simulink model "dcdc_joint"  (R2020b)
settings: Solver=VariableStepAuto  StartTime=0.0  StopTime=0.4  FixedStep=t_step  MaxStep=1e-6  RelTol=1e-3
undefined symbols (not defined in the file): Cb, Ion, Lb, Lithium, t_step
libraries: powerlib x19, powerlib_meascontrol x5, electricdrivelib x1
settings Model: Creator=Chuanyue Li  LastModifiedBy=c2107789
settings SolverCC: ZeroCrossAlgorithm=Adaptive
settings DataIOCC: ReturnWorkspaceOutputs=off
settings DebuggingCC: IgnoredZcDiagnostic=none  ArithmeticOperatorsInVariantConditions=warning
settings SFSimCC: SimUseLocalCustomCode=off  CustomCodeUndefinedFunction=UseInterfaceOnly
settings RTWCC: RTWUseLocalCustomCode=off

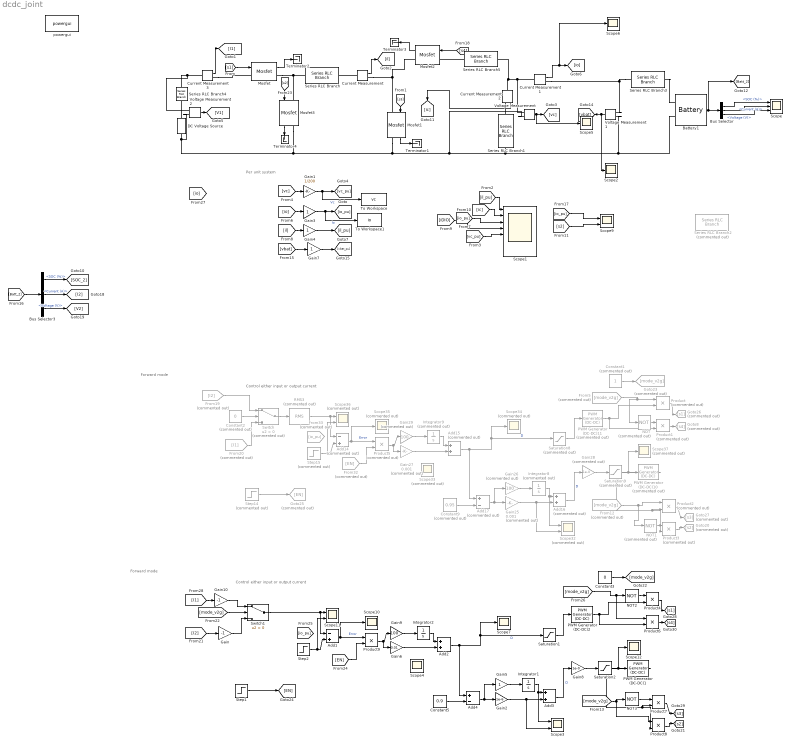
== system dcdc_joint ==
  note: Control either input or output current
  note: Per unit system
  note: Forward mode
  note: Control either input or output current
  note: Forward mode
  Add1 : Sum  Inputs=-+
  Add14 : Sum  Commented=on  Inputs=-+
  Add15 : Sum  Commented=on
  Add16 : Sum  Commented=on
  Add17 : Sum  Commented=on  Inputs=+-
  Add2 : Sum
  Add3 : Sum
  Add4 : Sum  Inputs=+-
  Battery1 : electricdrivelib/Extra Sources/Battery  BatType=Lithium-Ion  ShowTempParam=off  ThermalPreset=no  ShowAgeParam=off  NomV=380  NomQ=500  SOC=69.98  Batt_Tr=1  PresetModel=on  MaxQ=500  MinV=285  FullV=442.3151  Dis_rate=217.3913  R=0.0076  Normal_OP=452.1739  expZone="[410.5466      24.56522]"  current=[6.5 13 32.5]  Units=Time  Tci=20  NomT=20  T2=-30  MaxQ2=4.8  FullV2=7.1  Normal_OP2=5.655  expZone2="[6.58           1]"  Rca=0.6  ti=2000  Dp=0  Neq0=0  Tsim=1e6  Ta1=25  Qeol=5.4*0.9  Reol=0.013333*1.2  Char_age=[2.3478, 3]  Dis_age=[2.3478, 10]  N1=1500  N2=10500  N3=1000  N4=1400  Ta2=45  N5=950
  Bus Selector : BusSelector  OutputSignals=SOC (%),Current (A),Voltage (V)
  Bus Selector3 : BusSelector  OutputSignals=SOC (%),Current (A),Voltage (V)
  Constant1 : Constant  Commented=on
  Constant2 : Constant  Commented=on  Value=0
  Constant3 : Constant  Value=0
  Constant5 : Constant  Value=0.9
  Constant9 : Constant  Commented=on  Value=0.95
  Current Measurement{,1..3} (4 alike) : powerlib/Measurements/Current Measurement  PhasorSimulation=off  OutputType=Complex  PSBequivalent=0
  DC Voltage Source : powerlib/Electrical Sources/DC Voltage Source  Amplitude=415  Measurements=None
  From12 : From  Commented=on  GotoTag=mode_v2g
  From19 : From  Commented=on  GotoTag=I2
  From20 : From  Commented=on  GotoTag=I1
  From32 : From  Commented=on  GotoTag=EN
  From33 : From  Commented=on  GotoTag=io_pu
  From5 : From  Commented=on  GotoTag=mode_v2g
  Gain : Gain  Gain=-1
  Gain1 : Gain  Gain=1/200
  Gain10 : Gain  Gain=-1
  Gain2 : Gain  Gain=1e-6
  Gain25 : Gain  Commented=on  Gain=0.001
  Gain26 : Gain  Commented=on  Gain=100
  Gain27 : Gain  Commented=on  Gain=0.001
  Gain28 : Gain  Commented=on  Gain=1e-0
  Gain29 : Gain  Commented=on  Gain=100
  Gain{3..5,7} (4 alike) : Gain
  Gain6 : Gain  Gain=0.01
  Gain8 : Gain  Gain=1e-0
  Gain9 : Gain  Gain=100
  Goto20 : Goto  Commented=on  GotoTag=s2
  Goto23 : Goto  Commented=on  GotoTag=mode_v2g
  Goto25 : Goto  Commented=on  GotoTag=EN
  Goto26 : Goto  Commented=on  GotoTag=s1
  Goto27 : Goto  Commented=on  GotoTag=s3
  Goto8 : Goto  Commented=on  GotoTag=s4
  Integrator1 : Integrator  LimitOutput=on  UpperSaturationLimit=1  LowerSaturationLimit=0
  Integrator2 : Integrator  LimitOutput=on  UpperSaturationLimit=2  LowerSaturationLimit=0
  Integrator8 : Integrator  Commented=on  LimitOutput=on  UpperSaturationLimit=1  LowerSaturationLimit=0
  Integrator9 : Integrator  Commented=on  LimitOutput=on  UpperSaturationLimit=2  LowerSaturationLimit=0
  Mosfet : powerlib/Power Electronics/Mosfet  Ron=0.1  Lon=0  Rd=0.01  Vfd=0  IC=0  Rs=1e5  Cs=inf  Measurements=on
  Mosfet1 : powerlib/Power Electronics/Mosfet  Ron=0.01  Lon=0  Rd=0.01  Vfd=0  IC=0  Rs=1e5  Cs=inf  Measurements=on
  Mosfet2 : powerlib/Power Electronics/Mosfet  Ron=0.1  Lon=0  Rd=0.01  Vfd=0  IC=0  Rs=1e5  Cs=inf  Measurements=on
  Mosfet3 : powerlib/Power Electronics/Mosfet  Ron=0.1  Lon=0  Rd=0.01  Vfd=0  IC=0  Rs=1e5  Cs=inf  Measurements=on
  NOT : Logic  Commented=on  Operator=NOT  IconShape=distinctive  AllPortsSameDT=off  OutDataTypeStr=boolean
  NOT1 : Logic  Commented=on  Operator=NOT  IconShape=distinctive  AllPortsSameDT=off  OutDataTypeStr=boolean
  NOT2 : Logic  Operator=NOT  IconShape=distinctive  AllPortsSameDT=off  OutDataTypeStr=boolean
  NOT3 : Logic  Operator=NOT  IconShape=distinctive  AllPortsSameDT=off  OutDataTypeStr=boolean
  PWM Generator (DC-DC)1 : powerlib_meascontrol/Pulse & Signal Generators/PWM Generator (DC-DC)  Fsw=s_fre  Ts=0
  PWM Generator (DC-DC)10 : powerlib_meascontrol/Pulse & Signal Generators/PWM Generator (DC-DC)  Commented=on  Fsw=s_fre  Ts=0
  PWM Generator (DC-DC)11 : powerlib_meascontrol/Pulse & Signal Generators/PWM Generator (DC-DC)  Commented=on  Fsw=s_fre  Ts=0
  PWM Generator (DC-DC)2 : powerlib_meascontrol/Pulse & Signal Generators/PWM Generator (DC-DC)  Fsw=s_fre  Ts=0
  Product{,1..3,5} (5 alike) : Product  Commented=on
  Product{4,6..9} (5 alike) : Product
  RMS3 : powerlib_meascontrol/Measurements/RMS  Commented=on  TrueRMS=on  Freq=s_fre  RMSInit=0  Ts=0
  Saturation1 : Saturate  UpperLimit=1  LowerLimit=0
  Saturation2 : Saturate  UpperLimit=0.8  LowerLimit=0
  Saturation8 : Saturate  Commented=on  UpperLimit=1  LowerLimit=0
  Saturation9 : Saturate  Commented=on  UpperLimit=0.8  LowerLimit=0
  Scope : Scope  NumInputPorts=3
  Scope1 : Scope  NumInputPorts=8
  Scope{2,4..7,10,12} (7 alike) : Scope
  Scope11 : Scope  NumInputPorts=2
  Scope3 : Scope  NumInputPorts=2
  Scope32 : Scope  Commented=on  NumInputPorts=2
  Scope{33..35,37} (4 alike) : Scope  Commented=on
  Scope36 : Scope  Commented=on  NumInputPorts=2
  Scope9 : Scope  NumInputPorts=2
  Series RLC Branch : powerlib/Elements/Series RLC Branch  LConnTagsString=__new0  RConnTagsString=__new0  BranchType=L  Resistance=1  Inductance=Lb/100  SetiL0=off  InitialCurrent=0  Capacitance=1e-6  Setx0=off  InitialVoltage=0  Measurements=None
  Series RLC Branch1 : powerlib/Elements/Series RLC Branch  LConnTagsString=__new0  RConnTagsString=__new0  BranchType=C  Resistance=1  Inductance=1e-3  SetiL0=off  InitialCurrent=0  Capacitance=Cb  Setx0=off  InitialVoltage=0  Measurements=None
  Series RLC Branch2 : powerlib/Elements/Series RLC Branch  Commented=on  LConnTagsString=__new0  RConnTagsString=__new0  BranchType=L  Resistance=1  Inductance=Lb/100  SetiL0=off  InitialCurrent=0  Capacitance=1e-6  Setx0=off  InitialVoltage=0  Measurements=None
  Series RLC Branch3 : powerlib/Elements/Series RLC Branch  LConnTagsString=__new0  RConnTagsString=__new0  BranchType=R  Resistance=1  Inductance=Lb/100  SetiL0=off  InitialCurrent=0  Capacitance=1e-6  Setx0=off  InitialVoltage=0  Measurements=None
  Series RLC Branch4 : powerlib/Elements/Series RLC Branch  LConnTagsString=__new0  RConnTagsString=__new0  BranchType=R  Resistance=1e-3  Inductance=1e-3  SetiL0=off  InitialCurrent=0  Capacitance=Cb  Setx0=off  InitialVoltage=0  Measurements=None
  Series RLC Branch5 : powerlib/Elements/Series RLC Branch  LConnTagsString=__new0  RConnTagsString=__new0  BranchType=L  Resistance=1  Inductance=Lb/100  SetiL0=off  InitialCurrent=0  Capacitance=1e-6  Setx0=off  InitialVoltage=0  Measurements=None
  Step1 : Step  Time=0.025  SampleTime=0
  Step14 : Step  Commented=on  Time=0.025  SampleTime=0
  Step15 : Step  Commented=on  Before=10  After=11  SampleTime=0
  Step2 : Step  Before=30  After=11  SampleTime=0
  Switch : Switch  Commented=on  Criteria=u2 > Threshold
  Switch1 : Switch  Criteria=u2 > Threshold
  Terminator{1..4} (4 alike) : Terminator
  To Workspace : ToWorkspace  VariableName=vc  SaveFormat=Timeseries  SampleTime=-1
  To Workspace1 : ToWorkspace  VariableName=io  SaveFormat=Timeseries  SampleTime=-1
  Voltage Measurement : powerlib/Measurements/Voltage Measurement  PhasorSimulation=off  OutputType=Complex  PSBequivalent=0
  Voltage Measurement1 : powerlib/Measurements/Voltage Measurement  PhasorSimulation=off  OutputType=Complex  PSBequivalent=0
  Voltage Measurement2 : powerlib/Measurements/Voltage Measurement  PhasorSimulation=off  OutputType=Complex  PSBequivalent=0
  powergui : powerlib/powergui  Priority=1  SimulationMode=Continuous  SampleTime=t_step*10  frequency=60  Iterations=50  frequencyindice=0  Pbase=100e6  ErrMax=1e-4  UnitsV=kV  UnitsW=MW  buscounter=0  FunctionMessages=off  echomessages=off  EnableUseOfTLC=off  CurrentSourceSwitches=off  DisableSnubberDevices=off  DisableRonSwitches=off  DisableVfSwitches=off  DisplayEquations=off  AutomaticDiscreteSolvers=off  SolverType=Tustin/Backward Euler (TBE)  Interpol=off  ExternalGateDelay=off  methode=off  Ts=100  x0status=blocks  SPID=off  SwTol=0  HookPort=off  NonlinearTolerance=1e-4  nMaxIteration=100  ContinueOnMaxIteration=off  RestoreLinks=warning  ResistiveCurrentMeasurement=off  Frange=[0:2:500]  Ylog=off  Xlog=on  ShowGrid=off  save=off  variable=ZData  structure=0  ZoomFFT=off  StartTime=0.0  cycles=1  DisplayStyle=1  fundamental=60  FreqAxis=off  MaxFrequency=1000  frequencyindicesteady=1  RmsSteady=1  display=off
  wires:
  [s1] -> Mosfet/1
  [s3] -> Mosfet1/1
  Current Measurement/1 -> [il]
  Voltage Measurement/1 -> Scope5/1, [vc]
  [il_pu] -> Scope1/1
  [vc] -> Gain1/1
  Gain1/1 -> To Workspace/1, [vc_pu]  "Vc"
  Bus Selector/1 -> Scope/1  "<SOC (%)>"
  Bus Selector/2 -> Scope/2  "<Current (A)>"
  Bus Selector/3 -> Scope/3  "<Voltage (V)>"
  [io] -> Gain3/1
  Current Measurement1/1 -> Scope6/1, [io]
  Gain3/1 -> To Workspace1/1, [io_pu]  "Io"
  [io_pu] -> Scope1/3
  Gain4/1 -> [il_pu]
  [il] -> Gain4/1
  [iDIO] -> Scope1/4
  Current Measurement2/1 -> [ic]
  [ic] -> Scope1/2
  [vc_pu] -> Scope1/5
  Voltage Measurement1/1 -> Scope2/1, [vbat]
  [vbat] -> Gain7/1
  Gain7/1 -> [vbat_pu]
  Mosfet1/1 -> Terminator1/1
  Mosfet/1 -> Terminator2/1
  [io_pu] -> Scope9/1
  [s2] -> Scope9/2
  Mosfet2/1 -> Terminator3/1
  [s4] -> Mosfet2/1
  [s2] -> Mosfet3/1
  Mosfet3/1 -> Terminator4/1
  Add16/1 -> Gain28/1  "D"
  Gain26/1 -> Integrator8/1
  Gain25/1 -> Add16/2, Scope32/2
  Integrator8/1 -> Add16/1, Scope32/1
  Saturation8/1 -> PWM Generator (DC-DC)11/1
  Integrator9/1 -> Add15/1
  Add15/1 -> Saturation8/1, Scope34/1, Add17/1  "D"
  From32/1 -> Product5/2
  Product5/1 -> Gain29/1, Gain27/1
  Step14/1 -> Goto25/1
  Gain27/1 -> Add15/2
  Gain29/1 -> Integrator9/1
  Step15/1 -> Scope36/2, Add14/2
  Add14/1 -> Product5/1, Scope35/1  "Error"
  Saturation9/1 -> PWM Generator (DC-DC)10/1, Scope37/1
  Switch/1 -> RMS3/1
  PWM Generator (DC-DC)11/1 -> Product/2, Product1/2
  Gain28/1 -> Saturation9/1
  Constant9/1 -> Add17/2
  Add17/1 -> Gain25/1, Gain26/1
  Battery1/1 -> [Batt_2], Bus Selector/1
  [Batt_2] -> Bus Selector3/1
  Bus Selector3/3 -> [V2]  "<Voltage (V)>"
  Bus Selector3/2 -> [I2]  "<Current (A)>"
  Bus Selector3/1 -> [SOC_2]  "<SOC (%)>"
  From19/1 -> Switch/1
  From20/1 -> Switch/3
  Constant2/1 -> Switch/2
  Product/1 -> Goto26/1
  Product1/1 -> Goto8/1
  NOT/1 -> Product1/1
  NOT1/1 -> Product3/1
  Product3/1 -> Goto20/1
  From12/1 -> NOT1/1, Product2/1
  Product2/1 -> Goto27/1
  PWM Generator (DC-DC)10/1 -> Product3/2, Product2/2
  Constant1/1 -> Goto23/1
  From5/1 -> Product/1, NOT/1
  Current Measurement3/1 -> [I1]
  Voltage Measurement2/1 -> [V1]
  RMS3/1 -> Add14/1, Scope36/1
  Switch1/1 -> Scope11/1, Add1/1
  Constant3/1 -> [mode_v2g]
  PWM Generator (DC-DC)1/1 -> Product7/2, Product8/2
  Product7/1 -> [s3]
  Product8/1 -> [s2]
  [mode_v2g] -> Product8/1, NOT3/1
  [mode_v2g] -> NOT2/1, Product6/1
  Product6/1 -> [s4]
  Product4/1 -> [s1]
  [mode_v2g] -> Switch1/2
  [I2] -> Gain/1
  Add4/1 -> Gain5/1, Gain2/1
  Constant5/1 -> Add4/2
  Gain8/1 -> Saturation2/1
  PWM Generator (DC-DC)2/1 -> Product6/2, Product4/2
  Saturation2/1 -> Scope12/1, PWM Generator (DC-DC)1/1
  Add1/1 -> Scope10/1, Product9/1  "Error"
  Step2/1 -> Add1/2, Scope11/2
  Gain9/1 -> Integrator2/1
  Gain6/1 -> Add2/2
  Step1/1 -> [EN]
  Product9/1 -> Gain6/1, Gain9/1
  [EN] -> Product9/2
  Add2/1 -> Add4/1, Scope7/1, Saturation1/1  "D"
  Integrator2/1 -> Add2/1
  Saturation1/1 -> PWM Generator (DC-DC)2/1
  Integrator1/1 -> Scope3/1, Add3/1
  Gain2/1 -> Scope3/2, Add3/2
  Gain5/1 -> Integrator1/1
  Add3/1 -> Gain8/1  "D"
  NOT2/1 -> Product4/1
  NOT3/1 -> Product7/1
  Gain/1 -> Switch1/3
  Gain10/1 -> Switch1/1
  [I1] -> Gain10/1
  connections:
  Mosfet/RConn1 -- Mosfet3/LConn1 -- Series RLC Branch/LConn1
  Current Measurement/LConn1 -- Series RLC Branch/RConn1
  Current Measurement2/RConn1 -- Series RLC Branch1/LConn1
  Battery1/LConn2 -- Voltage Measurement/LConn2 -- Voltage Measurement2/LConn2 -- DC Voltage Source/LConn1 -- Mosfet3/RConn1 -- Mosfet1/RConn1 -- Series RLC Branch1/RConn1 -- Voltage Measurement1/LConn2
  Mosfet1/LConn1 -- Mosfet2/RConn1 -- Current Measurement/RConn1
  DC Voltage Source/RConn1 -- Series RLC Branch4/RConn1
  Series RLC Branch3/LConn1 -- Current Measurement1/RConn1 -- Voltage Measurement1/LConn1
  Current Measurement1/LConn1 -- Voltage Measurement/LConn1 -- Current Measurement2/LConn1 -- Series RLC Branch5/RConn1
  Current Measurement3/RConn1 -- Mosfet/LConn1
  Series RLC Branch4/LConn1 -- Voltage Measurement2/LConn1 -- Current Measurement3/LConn1
  Series RLC Branch5/LConn1 -- Mosfet2/LConn1
  Series RLC Branch3/RConn1 -- Battery1/LConn1
